simulink model "DB"  (R2024b)
settings: Solver=VariableStepAuto  StartTime=0.0  StopTime=100.0  RelTol=1e-3
values from neighbouring files (symbols this model uses):
  Gp_z = c2d(Gp,T_vz)    [main.m]
  P = [1, p1, p2, p3]    [dB_controller.m]    (also in main.m = P_nolimit)
  Q = [q0, q1, q2, q3]    [dB_controller.m]    (also in main.m = Q_nolimit)
settings Model: Creator=egoru  LastModifiedBy=egoru

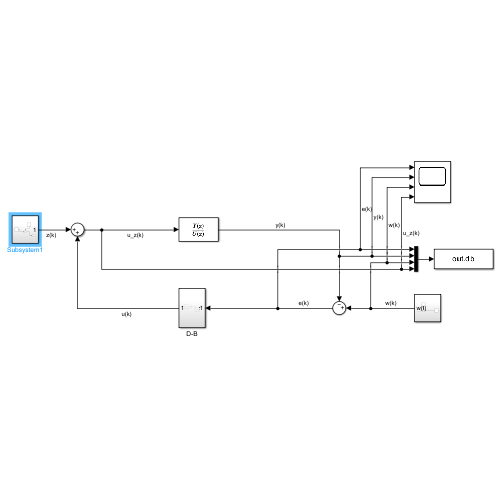
[thumbnail: Simulink's stored preview of the top-level diagram]
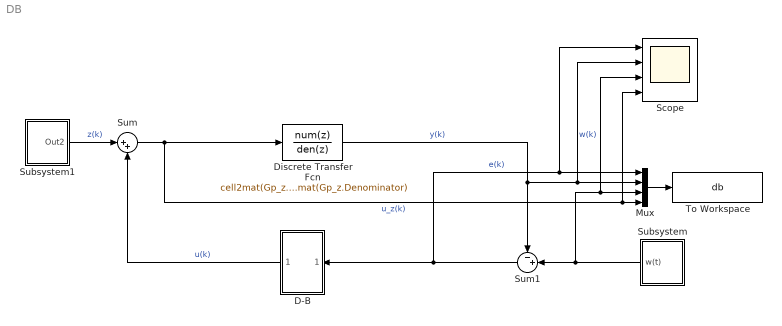
== system DB ==
  D-B : Subsystem
  Discrete Transfer Fcn : DiscreteTransferFcn  Numerator=cell2mat(Gp_z.Numerator)  Denominator=cell2mat(Gp_z.Denominator)
  Mux : Mux
  Scope : Scope  NumInputPorts=4
  Subsystem : Subsystem
  Subsystem1 : Subsystem
  Sum : Sum  Inputs=|++
  Sum1 : Sum  Inputs=-+|
  To Workspace : ToWorkspace  VariableName=db  SaveFormat=Timeseries  SampleTime=-1
  wires:
  Mux/1 -> To Workspace/1
  Discrete Transfer Fcn/1 -> Scope/2, Mux/2, Sum1/1  "y(k)"
  Sum1/1 -> D-B/1(In1), Scope/1, Mux/1  "e(k)"
  D-B/1(Out1) -> Sum/2  "u(k)"
  Subsystem/1(w(t)) -> Scope/3, Mux/3, Sum1/2  "w(k)"
  Sum/1 -> Discrete Transfer Fcn/1, Scope/4, Mux/4  "u_z(k)"
  Subsystem1/1(Out2) -> Sum/1  "z(k)"

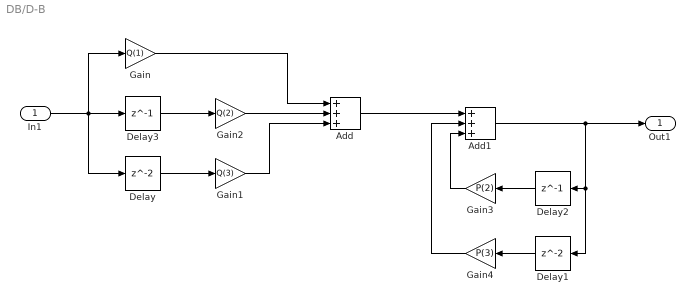
== system DB/D-B ==
  In1 : Inport
  Add : Sum  Inputs=+++
  Add1 : Sum  Inputs=+++
  Delay : Delay
  Delay1 : Delay
  Delay2 : Delay  DelayLength=1
  Delay3 : Delay  DelayLength=1
  Gain : Gain  Gain=Q(1)
  Gain1 : Gain  Gain=Q(3)
  Gain2 : Gain  Gain=Q(2)
  Gain3 : Gain  Gain=P(2)
  Gain4 : Gain  Gain=P(3)
  Out1 : Outport
  wires:
  Gain2/1 -> Add/2
  Gain1/1 -> Add/3
  Gain/1 -> Add/1
  In1/1 -> Delay/1, Delay3/1, Gain/1
  Add/1 -> Add1/1
  Add1/1 -> Out1/1, Delay1/1, Delay2/1
  Gain4/1 -> Add1/2
  Gain3/1 -> Add1/3
  Delay2/1 -> Gain3/1
  Delay1/1 -> Gain4/1
  Delay3/1 -> Gain2/1
  Delay/1 -> Gain1/1

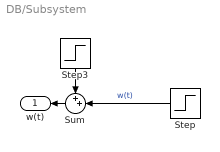
== system DB/Subsystem ==
  Step : Step  Time=10  SampleTime=0
  Step3 : Step  Time=70  After=-0.2  SampleTime=0
  Sum : Sum  Inputs=++|
  w(t) : Outport
  wires:
  Step3/1 -> Sum/1
  Step/1 -> Sum/2  "w(t)"
  Sum/1 -> w(t)/1

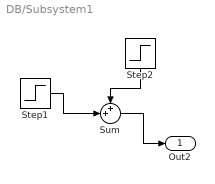
== system DB/Subsystem1 ==
  Step1 : Step  Time=30  After=0.02  SampleTime=0
  Step2 : Step  Time=40  After=-0.02  SampleTime=0
  Sum : Sum  Inputs=++|
  Out2 : Outport
  wires:
  Step2/1 -> Sum/1
  Step1/1 -> Sum/2
  Sum/1 -> Out2/1
